simulink model "SMC_Asintotico"  (R2026b)
settings Model: Creator=Yahoff  LastModifiedBy=Yahoff

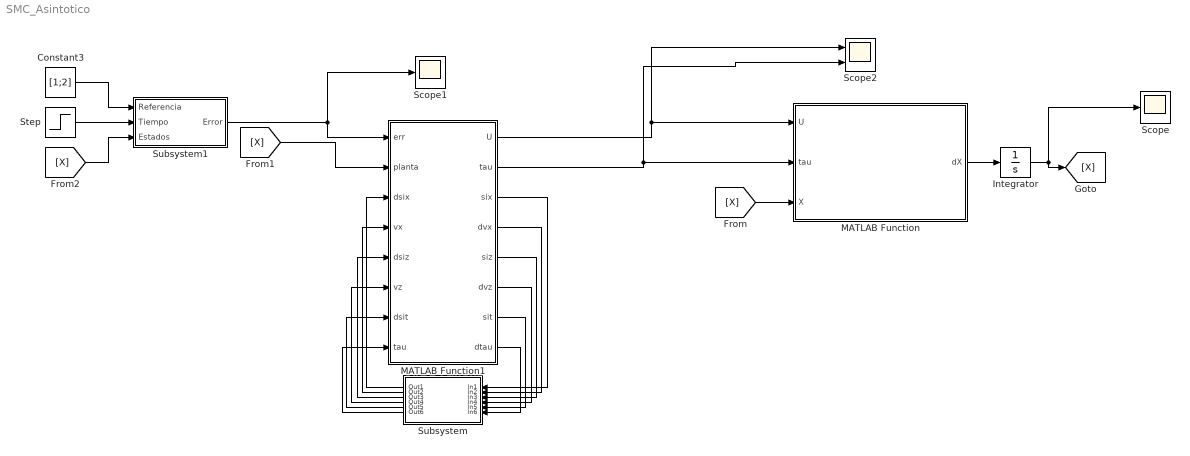
== system SMC_Asintotico ==
  Constant3 : Constant  Value=[1;2]
  Integrator : Integrator  InitialCondition=[0;0;0;0;0;0]
  MATLAB Function : MATLAB Function  TreatAsAtomicUnit=on
  MATLAB Function1 : MATLAB Function  TreatAsAtomicUnit=on
  Scope : Scope
      settings: ActiveDisplayYMinimum=-0.2507379151372866  ActiveDisplayYMaximum=2.25664123623558
  Scope1 : Scope
      settings: ActiveDisplayYMinimum=-0.13405317784249143  ActiveDisplayYMaximum=0.41916600704598622
  Scope2 : Scope  NumInputPorts=2
      settings: ActiveDisplayYMinimum=-2.5493283018714115  ActiveDisplayYMaximum=11.750334039297517  DataLoggingVariableName=ScopeData2
  Step : Step  SampleTime=0
  Subsystem : Subsystem
  Subsystem1 : Subsystem
  wires:
  MATLAB Function/1(dX) -> Integrator/1
  Integrator/1 -> [X], Scope/1
  [X] -> MATLAB Function/3(X)
  [X] -> MATLAB Function1/2(planta)
  MATLAB Function1/1(U) -> MATLAB Function/1(U), Scope2/1
  MATLAB Function1/2(tau) -> Scope2/2, MATLAB Function/2(tau)
  [X] -> Subsystem1/3(Estados)
  Constant3/1 -> Subsystem1/1(Referencia)
  Step/1 -> Subsystem1/2(Tiempo)
  Subsystem1/1(Error) -> Scope1/1, MATLAB Function1/1(err)
  MATLAB Function1/3(six) -> Subsystem/1(In1)
  MATLAB Function1/4(dvx) -> Subsystem/2(In2)
  MATLAB Function1/5(siz) -> Subsystem/3(In3)
  MATLAB Function1/6(dvz) -> Subsystem/4(In4)
  MATLAB Function1/7(sit) -> Subsystem/5(In5)
  MATLAB Function1/8(dtau) -> Subsystem/6(In6)
  Subsystem/1(Out1) -> MATLAB Function1/3(dsix)
  Subsystem/2(Out2) -> MATLAB Function1/4(vx)
  Subsystem/3(Out3) -> MATLAB Function1/5(dsiz)
  Subsystem/4(Out4) -> MATLAB Function1/6(vz)
  Subsystem/5(Out5) -> MATLAB Function1/7(dsit)
  Subsystem/6(Out6) -> MATLAB Function1/8("tau ")

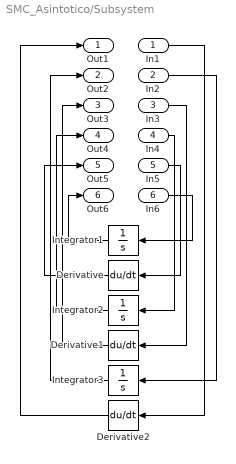
== system SMC_Asintotico/Subsystem ==
  In1 : Inport
  In2 : Inport  Port=2
  In3 : Inport  Port=3
  In4 : Inport  Port=4
  In5 : Inport  Port=5
  In6 : Inport  Port=6
  Derivative : Derivative
  Derivative1 : Derivative
  Derivative2 : Derivative
  Integrator1 : Integrator
  Integrator2 : Integrator
  Integrator3 : Integrator
  Out1 : Outport
  Out2 : Outport  Port=2
  Out3 : Outport  Port=3
  Out4 : Outport  Port=4
  Out5 : Outport  Port=5
  Out6 : Outport  Port=6
  wires:
  In5/1 -> Derivative/1
  Integrator1/1 -> Out6/1
  In3/1 -> Derivative1/1
  In4/1 -> Integrator2/1
  In6/1 -> Integrator1/1
  In1/1 -> Derivative2/1
  In2/1 -> Integrator3/1
  Derivative/1 -> Out5/1
  Integrator2/1 -> Out4/1
  Derivative1/1 -> Out3/1
  Integrator3/1 -> Out2/1
  Derivative2/1 -> Out1/1

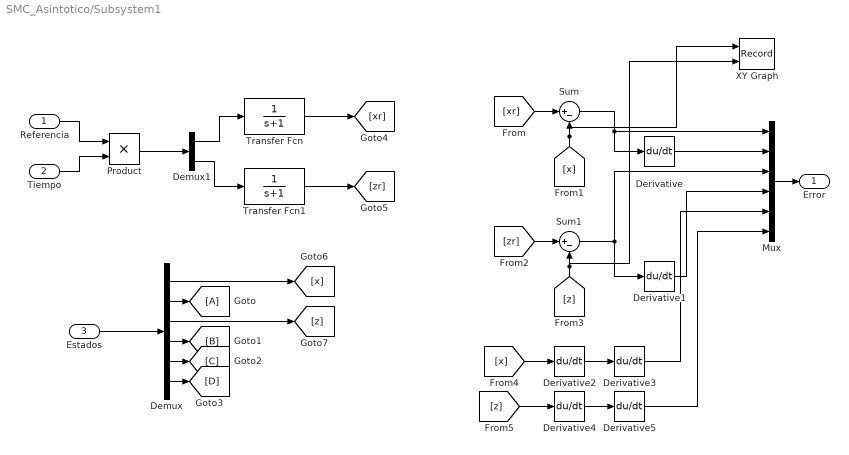
== system SMC_Asintotico/Subsystem1 ==
  Referencia : Inport
  Tiempo : Inport  Port=2
  Estados : Inport  Port=3
  Demux : Demux  Outputs=6
  Demux1 : Demux  Outputs=2
  Derivative{,1..5} (6 alike) : Derivative
  Goto : Goto
  Mux : Mux  Inputs=6
  Product : Product
  Sum : Sum  Inputs=|+-
  Sum1 : Sum  Inputs=|+-
  Transfer Fcn : TransferFcn  Denominator=[1 1]
  Transfer Fcn1 : TransferFcn  Denominator=[1 1]
  XY Graph : Record  NumPorts=2.0  FileSettingsInternal="{\"entries\":[{\"content\":{\"excelSettings\":{\"content\":{},\"type\":\"Streamout.ExcelSettings\"},\"parquetSettings\":{\"content\":{},\"type\":\"Streamout.ParquetSettings\"}},\"type\":\"Streamout.FileSettingStorage\",\"uuid\":\"\"}],\"packageUris\":[\"http:\\/\\/schema.mathworks.com\\/mf0\\/streamout_blocks\\/R2020a\"],\"version\":\"1.0\"}"  FrameSettings=[0, 0]  Layout=[1 1]  SignalsInternal="{\"entries\":[{\"content\":{\"signals\":[{\"content\":{\"blockPath\":[],\"dimensions\":[1],\"domain\":\"\",\"lineColor\":\"#a2142f\",\"plots\":[ 1 ],\"port\":1,\"sid\":[\"\"],\"signalID\":1,\"signalName\":\"From1\"},\"type\":\"RecordBlkView.Signal\",\"uuid\":\"\"},{\"content\":{\"blockPath\":[],\"dimensions\":[1],\"domain\":\"\",\"lineColor\":\"#139fff\",\"plots\":[ 1 ],\"port\":2,\"sid\":[\"\"],\"signalID\":2,\"signalName\":\"From3\"},\"type\":\"RecordBlkView.Signal\",\"uuid\":\"\"}]},\"type\":\"RecordBlkView.InputSignals\",\"uuid\":\"\"}],\"packageUris\":[\"http:\\/\\/schema.mathworks.com\\/mf0\\/streamout_blocks\\/R2020a\"],\"version\":\"1.0\"}"  VisualizationBindings="{\"xyplotplugin\":{\"info\":[{\"series\":[{\"bindingParametersList\":[{\"parameter\":\"X-Axis\",\"signalID\":1,\"signalName\":\"From1\"},{\"parameter\":\"Y-Axis\",\"signalID\":2,\"signalName\":\"From3\"}],\"seriesID\":0}],\"subplotID\":1}]}}"  CompatibilityTag=XY
  Error : Outport
  wires:
  Demux/3 -> [z]
  Demux/1 -> [x]
  Demux/5 -> [C]
  Demux/6 -> [D]
  Estados/1 -> Demux/1
  Demux/2 -> Goto/1
  Demux/4 -> [B]
  Referencia/1 -> Product/1
  Tiempo/1 -> Product/2
  Product/1 -> Demux1/1
  Demux1/2 -> Transfer Fcn1/1
  Demux1/1 -> Transfer Fcn/1
  Transfer Fcn/1 -> [xr]
  Transfer Fcn1/1 -> [zr]
  [xr] -> Sum/1
  [x] -> XY Graph/1, Sum/2
  [zr] -> Sum1/1
  [z] -> XY Graph/2, Sum1/2
  Sum/1 -> Derivative/1, Mux/1
  Sum1/1 -> Mux/3, Derivative1/1
  Derivative/1 -> Mux/2
  Derivative1/1 -> Mux/4
  Mux/1 -> Error/1
  Derivative2/1 -> Derivative3/1
  Derivative4/1 -> Derivative5/1
  [x] -> Derivative2/1
  [z] -> Derivative4/1
  Derivative3/1 -> Mux/5
  Derivative5/1 -> Mux/6

== matlab function SMC_Asintotico/MATLAB Function1 ==
  data: err input; U output; planta input; tau output; dsix input; six output; vx input; dvx output; dsiz input; vz input; dsit input; tau input; siz output; dvz output; sit output; dtau output
function [U, tau, six , dvx , siz , dvz ,sit, dtau] = control(err, planta,dsix,vx , dsiz , vz , dsit , tau)

    p = 1; g = 9.81;
    kth = 100; kom =50;

    k=4;%4
    m=1;%1
    l=2;%2
    n=1;%1

    ex = err(1);
    dex = err(2);
    ez = err(3);   
    dez = err(4);
    xrdd=err(5);
    zrdd=err(6);

    x     = planta(1);
    xdot  = planta(2);
    z     = planta(3);
    zdot  = planta(4);
    th    = planta(5);
    thdot = planta(6);

    six = dex + n*ex;
    Sx  = dsix + n*six;
    dvx = -n*m*xdot - (m+n)*vx + k*sign(Sx);
   
    siz = dez + n*ez;
    Sz  = dsiz+ n*siz;
    dvz = -n*m*zdot - (m+n)*vz + k*sign(Sz);

    U   = p*sqrt(vx^2 + (vz+g)^2);
    thd = atan2(-vx, vz+g);

    e = th - thd;
    de = thdot;

    j = 20;
    b = 10;
    d = 10;

    sit = de + b*e;
    St  = dsit + b*sit;
    dtau = -b*d*thdot -(b+d)*tau - j*sign(St);
end



function y = sat(u)
if u > 1
    y = 1;
elseif u < -1
    y = -1;
else
    y = u;
end
end

== matlab function SMC_Asintotico/MATLAB Function ==
  data: U input; dX output; tau input; X input
function dX = planta(U, tau, X)

    m = 1; J = 1; g = 9.81;
    kth = 30; kom = 12;

    x     = X(1);
    xdot  = X(2);
    z     = X(3);
    zdot  = X(4);
    th    = X(5);
    thdot = X(6);

    xdd  = -(U/m)*sin(th);
    zdd  =  (U/m)*cos(th) - g;
    thdd =  tau/J;

    dX = [xdot; xdd; zdot; zdd; thdot; thdd];
